simulink model "bh_compare_SM_vs_HAND_quad_and_spin_props"  (R2021b)
settings: Solver=ode23t  StartTime=0.0  StopTime=200  FixedStep=0.001  RelTol=1e-5  EnableMultiTasking=on
undefined symbols (not defined in the file or in its folder): P_elec, P_mot, P_one_prop, P_rot, P_veh, P_veh_no_props, sigbuilder_block, X, xme_dot_0, Y, Z
libraries: fl_lib x85, simulink_extras x40, nesl_utility x35, slpidlib x24, bh_6dof_LIBRARY x24, sm_lib x23, fl_ps_legacy_lib x7, simulink x2
(part 2 of 6)

== system bh_compare_SM_vs_HAND_quad_and_spin_props/XYZ CMD_LIMITS1 ==
  XYZ_in : Inport
  Bus Creator : BusCreator  Inputs=3
  Demux : Demux  Outputs=2
  Demux1 : Demux  Outputs=2
  Mux1 : Mux  Inputs=2
  Mux2 : Mux  Inputs=2
  Mux3 : Mux  Inputs=2
  Mux4 : Mux  Inputs=3
  Rate Limiter : RateLimiter  RisingSlewLimit=2  FallingSlewLimit=-2
      settings: AttributesFormatString=|
      | Rising_rate = %<RisingSlewLimit>
      | Falling_rate = %<FallingSlewLimit>
  Rate Limiter1 : RateLimiter  RisingSlewLimit=3  FallingSlewLimit=-3
      settings: AttributesFormatString=|
      | Rising_rate = %<RisingSlewLimit>
      | Falling_rate = %<FallingSlewLimit>
  Rate Limiter2 : RateLimiter  RisingSlewLimit=3  FallingSlewLimit=-3
      settings: AttributesFormatString=|
      | Rising_rate = %<RisingSlewLimit>
      | Falling_rate = %<FallingSlewLimit>
  Reshape : Reshape  OutputDimensionality=Column vector (2-D)
  Saturation : Saturate  UpperLimit=500  LowerLimit=0
      settings: AttributesFormatString=|
      | MAX =    %<UpperLimit>
      | MIN = %<LowerLimit>
  Saturation1 : Saturate  UpperLimit=500  LowerLimit=-500
      settings: AttributesFormatString=|
      | MAX =    %<UpperLimit>
      | MIN = %<LowerLimit>
  Saturation2 : Saturate  UpperLimit=500  LowerLimit=-500
      settings: AttributesFormatString=|
      | MAX =    %<UpperLimit>
      | MIN = %<LowerLimit>
  Selector : Selector  InputPortWidth=3  IndexOptions=Index vector (dialog)  Indices=3  OutputSizes=1
  Selector1 : Selector  InputPortWidth=3  IndexOptions=Index vector (dialog)  Indices=[1 2]  OutputSizes=1
  Unit Delay : UnitDelay  SampleTime=0.01  HasFrameUpgradeWarning=on
  Unit Delay1 : UnitDelay  SampleTime=0.01  HasFrameUpgradeWarning=on
  ZXY_LIMITED : Scope  NumInputPorts=3
  prefilter : Subsystem  Commented=on  mask(Derivative Estimation){wn=2*pi*0.5, p=1}
      mask prompts: wn "Natural frequency, wn (rad/sec)"; p "Damping ratio, p"
      mask help:
      | A simple derivative estimator using a 2nd order representation between input and output.
      |
      | The integrators use a discrete FORWARd Euler rule, and a sample time needs to be specified.
      mask init:
      | str1 = sprintf('wn = %.2f', wn);
      | str2 = sprintf('p  = %.2f', p);
      | %str3 = sprintf('dt = %.2f', dt);
      | %str = char(str1,str2,str3);
      | %str3 = sprintf('dt = %.2f', dt);
      | str = char(str1,str2);
      mask Display: disp(str)
  XYZ : Outport  VectorParamsAs1DForOutWhenUnconnected=off
  CMD_BUS : Outport  Port=2  VectorParamsAs1DForOutWhenUnconnected=off
  wires:
  Selector1/1 -> Demux1/1, Unit Delay1/1
  Demux/1 -> Rate Limiter1/1
  Demux/2 -> Rate Limiter2/1
  Saturation1/1 -> [X]
  Saturation2/1 -> [Y]
  Mux4/1 -> Reshape/1
  Selector/1 -> Mux1/1, Unit Delay/1
  Rate Limiter/1 -> Saturation/1
  Unit Delay/1 -> Rate Limiter/1
  Unit Delay1/1 -> Demux/1
  Rate Limiter1/1 -> Saturation1/1
  Rate Limiter2/1 -> Saturation2/1
  [X] -> Mux4/1
  [Y] -> Mux4/2
  [Z] -> Mux4/3
  Saturation/1 -> [Z]
  [Z] -> Mux1/2
  [Y] -> Mux3/2
  Demux1/1 -> Mux2/1
  Demux1/2 -> Mux3/1
  [X] -> Mux2/2
  Mux1/1 -> ZXY_LIMITED/1  "Z"
  Mux2/1 -> ZXY_LIMITED/2  "X"
  Mux3/1 -> ZXY_LIMITED/3  "Y"
  Bus Creator/1 -> CMD_BUS/1
  [Y] -> Bus Creator/2  "Y"
  [X] -> Bus Creator/1  "X"
  [Z] -> Bus Creator/3  "Z"
  Reshape/1 -> XYZ/1
  XYZ_in/1 -> Selector1/1, Selector/1

== system bh_compare_SM_vs_HAND_quad_and_spin_props/a_circle1 ==
  Clock : Clock
  Clock1 : Clock
  Constant4 : Constant  Value=0  VectorParams1D=off
  Constant5 : Constant  Value=20  VectorParams1D=off
  Constant6 : Constant  Value=2  VectorParams1D=off
  Constant7 : Constant  VectorParams1D=off
  Constant8 : Constant  Value=0.05  VectorParams1D=off
  MATLAB Function : MATLAB Function  TreatAsAtomicUnit=on
  Mux1 : Mux  Inputs=3
  Reshape1 : Reshape  OutputDimensionality=Column vector (2-D)
  Reshape2 : Reshape  OutputDimensionality=Column vector (2-D)
  Signal Builder : Subsystem  Tag=STV Subsys  LoadFcn=sigbuilder_block('load');  StartFcn=sigbuilder_block('start');  StopFcn=sigbuilder_block('stop');  ClipboardFcn=sigbuilder_block('clipboard');  mask(Sigbuilder block){tuvar=[0:10]}
      mask help: Simulink:masks:SigbuilderBlock_MD
      mask init:
      | if ~strcmp(get_param(bdroot(gcbh),'SimulationStatus'),'stopped') tuvar = sigbuilder_block('maskInit'); end
      settings: CopyFcn=sigbuilder_block('copy');  DeleteFcn=sigbuilder_block('delete');  ModelCloseFcn=sigbuilder_block('modelClose');  PreSaveFcn=sigbuilder_block('preSave');  PauseFcn=sigbuilder_block('pause');  ContinueFcn=sigbuilder_block('continue');  NameChangeFcn=sigbuilder_block('namechange');  OpenFcn=sigbuilder_block('open',[437.6 199.2 550.4 400 ]);  CloseFcn=sigbuilder_block('close');
      mask Display: plot(0, 0, 100, 100,[2, 2, 32, 32, 2], [68, 8, 8, 68, 68],[32, 2], [38, 38], [32, 19, 2],[53, 60, 44], [32, 17, 17, 2],[16, 16, 31, 31]);txt = getActiveGroup(gcbh);text(2, 100, txt,'verticalAlignment', 'top');
  Subsystem : Subsystem
  Switch : Switch  Criteria=u2 > Threshold  Threshold=20
  Out1 : Outport  VectorParamsAs1DForOutWhenUnconnected=off
  wires:
  Switch/1 -> Out1/1
  MATLAB Function/1(XYZ) -> Reshape2/1
  Constant6/1 -> MATLAB Function/3(RADIUS)
  Constant7/1 -> MATLAB Function/4(ztgt)
  Subsystem/1(w_rad_psec) -> MATLAB Function/5(w)
  Constant5/1 -> MATLAB Function/2(t_to_start)
  Reshape1/1 -> Switch/3
  Constant4/1 -> Mux1/2
  Signal Builder/1(Signal 1) -> Mux1/1
  Signal Builder/2(Signal 2) -> Mux1/3
  Mux1/1 -> Reshape1/1
  Clock/1 -> Switch/2
  Clock1/1 -> MATLAB Function/1(t_clock)
  Constant8/1 -> Subsystem/1(RPS)
  Reshape2/1 -> Switch/1

== system bh_compare_SM_vs_HAND_quad_and_spin_props/CONT_SYS Force_Moment_CMDS/FM_CMD_LIMITS ==
  T_CMD : Inport
  TQ_Roll : Inport  Port=2
  TQ_Pitch : Inport  Port=3
  TQ_Yaw : Inport  Port=4
  Mux : Mux
  Saturation : Saturate  UpperLimit=4*P_one_prop.thrust_max  LowerLimit=0
      settings: AttributesFormatString=|
      | MAX =    %<UpperLimit>
      | MIN = %<LowerLimit>
  Saturation1 : Saturate  UpperLimit=2*P_one_prop.TQ_max  LowerLimit=-2*P_one_prop.TQ_max
      settings: AttributesFormatString=|
      | MAX =    %<UpperLimit>
      | MIN = %<LowerLimit>
  Saturation2 : Saturate  UpperLimit="P_one_prop.thrust_max *  P_veh.L_CG_to_mot"  LowerLimit="-P_one_prop.thrust_max *  P_veh.L_CG_to_mot"
      settings: AttributesFormatString=|
      | MAX =    %<UpperLimit>
      | MIN = %<LowerLimit>
  Saturation3 : Saturate  UpperLimit="P_one_prop.thrust_max *  P_veh.L_CG_to_mot"  LowerLimit="-P_one_prop.thrust_max *  P_veh.L_CG_to_mot"
      settings: AttributesFormatString=|
      | MAX =    %<UpperLimit>
      | MIN = %<LowerLimit>
  THRUST : Outport  VectorParamsAs1DForOutWhenUnconnected=off
  TQ_Roll_X : Outport  Port=2  VectorParamsAs1DForOutWhenUnconnected=off
  TQ_Pitch_Y : Outport  Port=3  VectorParamsAs1DForOutWhenUnconnected=off
  TQ_Yaw_Z : Outport  Port=4  VectorParamsAs1DForOutWhenUnconnected=off
  CMD_VEC : Outport  Port=5  VectorParamsAs1DForOutWhenUnconnected=off
  wires:
  TQ_Yaw/1 -> Saturation1/1
  T_CMD/1 -> Saturation/1
  TQ_Pitch/1 -> Saturation2/1
  TQ_Roll/1 -> Saturation3/1
  Saturation/1 -> [THRUST], THRUST/1
  Saturation3/1 -> [TQ_Roll_X], TQ_Roll_X/1
  Saturation2/1 -> [TQ_Pitch_Y], TQ_Pitch_Y/1
  Saturation1/1 -> [TQ_Yaw_Z], TQ_Yaw_Z/1
  Mux/1 -> CMD_VEC/1
  [THRUST] -> Mux/1
  [TQ_Roll_X] -> Mux/2
  [TQ_Pitch_Y] -> Mux/3
  [TQ_Yaw_Z] -> Mux/4

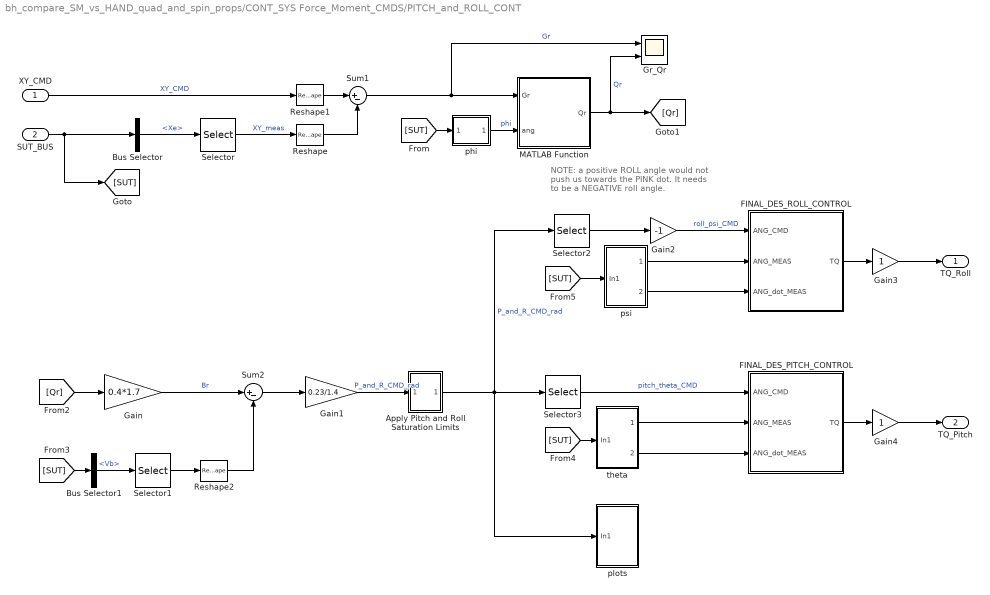
== system bh_compare_SM_vs_HAND_quad_and_spin_props/CONT_SYS Force_Moment_CMDS/PITCH_and_ROLL_CONT ==
  note: NOTE:  a positive ROLL angle would
      | not push us towards the PINK dot.  It
      | needs to be a NEGATIVE roll angle.
  XY_CMD : Inport
  SUT_BUS : Inport  Port=2
  Apply Pitch and Roll Saturation Limits : Subsystem
  Bus Selector : BusSelector  OutputSignals=Xe
  Bus Selector1 : BusSelector  OutputSignals=Vb
  FINAL_DES_PITCH_CONTROL : Subsystem
  FINAL_DES_ROLL_CONTROL : Subsystem
  Gain : Gain  Gain=0.4*1.7
  Gain1 : Gain  Gain=0.23/1.4
  Gain2 : Gain  Gain=-1
  Gain3 : Gain
  Gain4 : Gain
  Gr_Qr : Scope  NumInputPorts=2
  MATLAB Function : MATLAB Function  TreatAsAtomicUnit=on
  Reshape : Reshape  OutputDimensionality=Column vector (2-D)
  Reshape1 : Reshape  OutputDimensionality=Column vector (2-D)
  Reshape2 : Reshape  OutputDimensionality=Column vector (2-D)
  Selector : Selector  InputPortWidth=3  IndexOptions=Index vector (dialog)  Indices=[1 2]  OutputSizes=1
  Selector1 : Selector  InputPortWidth=3  IndexOptions=Index vector (dialog)  Indices=[1 2]  OutputSizes=1
  Selector2 : Selector  InputPortWidth=2  IndexOptions=Index vector (dialog)  Indices=2  OutputSizes=1
  Selector3 : Selector  InputPortWidth=2  IndexOptions=Index vector (dialog)  Indices=1  OutputSizes=1
  Sum1 : Sum  Inputs=|+-
  Sum2 : Sum  Inputs=|+-
  phi : Subsystem
  plots : Subsystem
  psi : Subsystem
  theta : Subsystem
  TQ_Roll : Outport  VectorParamsAs1DForOutWhenUnconnected=off
  TQ_Pitch : Outport  Port=2  VectorParamsAs1DForOutWhenUnconnected=off
  wires:
  Bus Selector/1 -> Selector/1  "<Xe>"
  Selector/1 -> Reshape/1  "XY_meas"
  SUT_BUS/1 -> Bus Selector/1, [SUT]
  XY_CMD/1 -> Reshape1/1  "XY_CMD"
  Reshape1/1 -> Sum1/1
  Reshape/1 -> Sum1/2
  Sum1/1 -> Gr_Qr/1, MATLAB Function/1(Gr)  "Gr"
  [SUT] -> phi/1(In1)
  phi/1(Out1) -> MATLAB Function/2(ang)  "phi"
  MATLAB Function/1(Qr) -> Gr_Qr/2, [Qr]  "Qr"
  [Qr] -> Gain/1
  Gain/1 -> Sum2/1  "Br"
  Bus Selector1/1 -> Selector1/1  "<Vb>"
  [SUT] -> Bus Selector1/1
  Selector1/1 -> Reshape2/1
  Reshape2/1 -> Sum2/2
  Sum2/1 -> Gain1/1
  [SUT] -> theta/1(In1)
  theta/1(Out1) -> FINAL_DES_PITCH_CONTROL/2(ANG_MEAS)
  theta/2(Out2) -> FINAL_DES_PITCH_CONTROL/3(ANG_dot_MEAS)
  Selector3/1 -> FINAL_DES_PITCH_CONTROL/1(ANG_CMD)  "pitch_theta_CMD"
  FINAL_DES_PITCH_CONTROL/1(TQ) -> Gain4/1
  Gain1/1 -> Apply Pitch and Roll Saturation Limits/1(In1)  "P_and_R_CMD_rad"
  Selector2/1 -> Gain2/1
  psi/1(Out1) -> FINAL_DES_ROLL_CONTROL/2(ANG_MEAS)
  psi/2(Out2) -> FINAL_DES_ROLL_CONTROL/3(ANG_dot_MEAS)
  [SUT] -> psi/1(In1)
  FINAL_DES_ROLL_CONTROL/1(TQ) -> Gain3/1
  Gain2/1 -> FINAL_DES_ROLL_CONTROL/1(ANG_CMD)  "roll_psi_CMD"
  Apply Pitch and Roll Saturation Limits/1(Out1) -> plots/1(In1), Selector3/1, Selector2/1  "P_and_R_CMD_rad"
  Gain3/1 -> TQ_Roll/1
  Gain4/1 -> TQ_Pitch/1

== system bh_compare_SM_vs_HAND_quad_and_spin_props/CONT_SYS Force_Moment_CMDS/YAW_CONT ==
  Yaw_CMD : Inport
  SUT_BUS : Inport  Port=2
  Bus Selector3 : BusSelector  OutputSignals=phi_theta_psi
  Bus Selector4 : BusSelector  OutputSignals=DOT_phi_theta_psi
  FINAL_DES_YAW_CONTROL_SYSTEM : Subsystem
  Selector2 : Selector  InputPortWidth=3  IndexOptions=Index vector (dialog)  Indices=1  OutputSizes=1
  Selector3 : Selector  InputPortWidth=3  IndexOptions=Index vector (dialog)  Indices=1  OutputSizes=1
  TQ_Yaw : Outport  VectorParamsAs1DForOutWhenUnconnected=off
  wires:
  Selector2/1 -> FINAL_DES_YAW_CONTROL_SYSTEM/2(YAW_MEAS)
  Yaw_CMD/1 -> FINAL_DES_YAW_CONTROL_SYSTEM/1(YAW_CMD)
  Selector3/1 -> FINAL_DES_YAW_CONTROL_SYSTEM/3(YAW_dot_MEAS)
  FINAL_DES_YAW_CONTROL_SYSTEM/1(TQ_YAW) -> TQ_Yaw/1  "TQ_Z_YAW"
  Bus Selector4/1 -> Selector3/1  "<DOT_phi_theta_psi>"
  Bus Selector3/1 -> Selector2/1  "<phi_theta_psi>"
  SUT_BUS/1 -> Bus Selector4/1, Bus Selector3/1

== system bh_compare_SM_vs_HAND_quad_and_spin_props/CONT_SYS Force_Moment_CMDS/Z_CONT ==
  Ze_CMD : Inport
  SUT_BUS : Inport  Port=2
  Bus Selector : BusSelector  OutputSignals=Xe
  Bus Selector2 : BusSelector  OutputSignals=Ve
  FINAL_DES_ALTITUDE_CONTROL_SYSTEM : Subsystem
  Selector : Selector  InputPortWidth=3  IndexOptions=Index vector (dialog)  Indices=3  OutputSizes=1
  Selector1 : Selector  InputPortWidth=3  IndexOptions=Index vector (dialog)  Indices=3  OutputSizes=1
  Ze_to_Altitude : bh_6dof_LIBRARY/MODELS/Ze_to_Altitude  SystemSampleTime=-1  VariantActivationTime=update diagram  Latency=0  AutoFrameSizeCalculation=off
  THRUST : Outport  VectorParamsAs1DForOutWhenUnconnected=off
  wires:
  Selector1/1 -> FINAL_DES_ALTITUDE_CONTROL_SYSTEM/3(Ze_dot_MEAS)
  Ze_to_Altitude/1 -> FINAL_DES_ALTITUDE_CONTROL_SYSTEM/2(Ze_MEAS)
  FINAL_DES_ALTITUDE_CONTROL_SYSTEM/1(THRUST) -> THRUST/1
  SUT_BUS/1 -> Bus Selector2/1, Bus Selector/1
  Ze_CMD/1 -> FINAL_DES_ALTITUDE_CONTROL_SYSTEM/1(Ze_CMD)
  Bus Selector2/1 -> Selector1/1  "<Ve>"
  Bus Selector/1 -> Selector/1  "<Xe>"
  Selector/1 -> Ze_to_Altitude/1

== system bh_compare_SM_vs_HAND_quad_and_spin_props/CONT_SYS Force_Moment_CMDS1/FM_CMD_LIMITS ==
  T_CMD : Inport
  TQ_Roll : Inport  Port=2
  TQ_Pitch : Inport  Port=3
  TQ_Yaw : Inport  Port=4
  Mux : Mux
  Saturation : Saturate  UpperLimit=4*P_one_prop.thrust_max  LowerLimit=0
      settings: AttributesFormatString=|
      | MAX =    %<UpperLimit>
      | MIN = %<LowerLimit>
  Saturation1 : Saturate  UpperLimit=2*P_one_prop.TQ_max  LowerLimit=-2*P_one_prop.TQ_max
      settings: AttributesFormatString=|
      | MAX =    %<UpperLimit>
      | MIN = %<LowerLimit>
  Saturation2 : Saturate  UpperLimit="P_one_prop.thrust_max *  P_veh.L_CG_to_mot"  LowerLimit="-P_one_prop.thrust_max *  P_veh.L_CG_to_mot"
      settings: AttributesFormatString=|
      | MAX =    %<UpperLimit>
      | MIN = %<LowerLimit>
  Saturation3 : Saturate  UpperLimit="P_one_prop.thrust_max *  P_veh.L_CG_to_mot"  LowerLimit="-P_one_prop.thrust_max *  P_veh.L_CG_to_mot"
      settings: AttributesFormatString=|
      | MAX =    %<UpperLimit>
      | MIN = %<LowerLimit>
  THRUST : Outport  VectorParamsAs1DForOutWhenUnconnected=off
  TQ_Roll_X : Outport  Port=2  VectorParamsAs1DForOutWhenUnconnected=off
  TQ_Pitch_Y : Outport  Port=3  VectorParamsAs1DForOutWhenUnconnected=off
  TQ_Yaw_Z : Outport  Port=4  VectorParamsAs1DForOutWhenUnconnected=off
  CMD_VEC : Outport  Port=5  VectorParamsAs1DForOutWhenUnconnected=off
  wires:
  TQ_Yaw/1 -> Saturation1/1
  T_CMD/1 -> Saturation/1
  TQ_Pitch/1 -> Saturation2/1
  TQ_Roll/1 -> Saturation3/1
  Saturation/1 -> [THRUST], THRUST/1
  Saturation3/1 -> [TQ_Roll_X], TQ_Roll_X/1
  Saturation2/1 -> [TQ_Pitch_Y], TQ_Pitch_Y/1
  Saturation1/1 -> [TQ_Yaw_Z], TQ_Yaw_Z/1
  Mux/1 -> CMD_VEC/1
  [THRUST] -> Mux/1
  [TQ_Roll_X] -> Mux/2
  [TQ_Pitch_Y] -> Mux/3
  [TQ_Yaw_Z] -> Mux/4

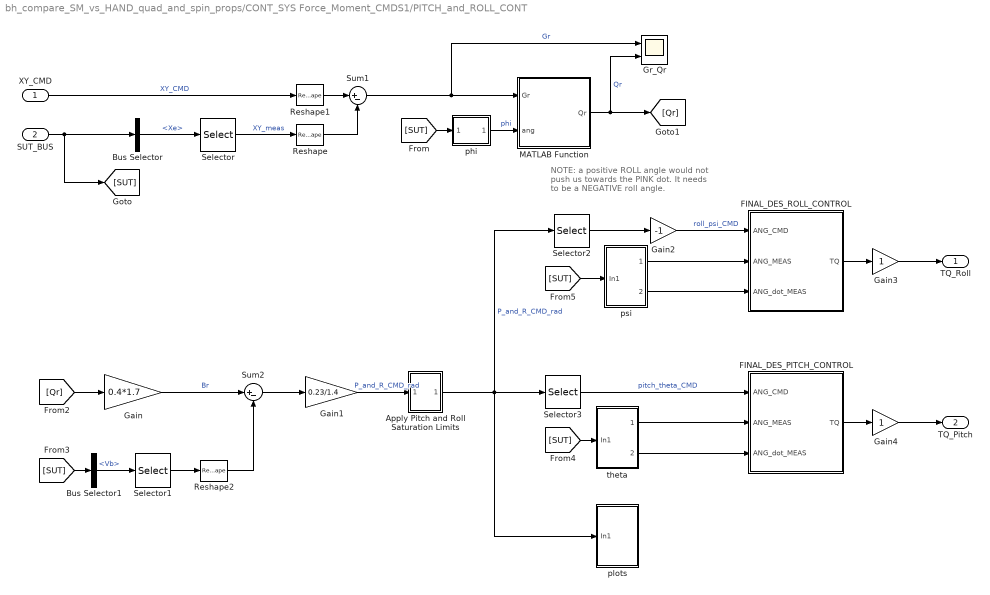
== system bh_compare_SM_vs_HAND_quad_and_spin_props/CONT_SYS Force_Moment_CMDS1/PITCH_and_ROLL_CONT ==
  note: NOTE:  a positive ROLL angle would
      | not push us towards the PINK dot.  It
      | needs to be a NEGATIVE roll angle.
  XY_CMD : Inport
  SUT_BUS : Inport  Port=2
  Apply Pitch and Roll Saturation Limits : Subsystem
  Bus Selector : BusSelector  OutputSignals=Xe
  Bus Selector1 : BusSelector  OutputSignals=Vb
  FINAL_DES_PITCH_CONTROL : Subsystem
  FINAL_DES_ROLL_CONTROL : Subsystem
  Gain : Gain  Gain=0.4*1.7
  Gain1 : Gain  Gain=0.23/1.4
  Gain2 : Gain  Gain=-1
  Gain3 : Gain
  Gain4 : Gain
  Gr_Qr : Scope  NumInputPorts=2
  MATLAB Function : MATLAB Function  TreatAsAtomicUnit=on
  Reshape : Reshape  OutputDimensionality=Column vector (2-D)
  Reshape1 : Reshape  OutputDimensionality=Column vector (2-D)
  Reshape2 : Reshape  OutputDimensionality=Column vector (2-D)
  Selector : Selector  InputPortWidth=3  IndexOptions=Index vector (dialog)  Indices=[1 2]  OutputSizes=1
  Selector1 : Selector  InputPortWidth=3  IndexOptions=Index vector (dialog)  Indices=[1 2]  OutputSizes=1
  Selector2 : Selector  InputPortWidth=2  IndexOptions=Index vector (dialog)  Indices=2  OutputSizes=1
  Selector3 : Selector  InputPortWidth=2  IndexOptions=Index vector (dialog)  Indices=1  OutputSizes=1
  Sum1 : Sum  Inputs=|+-
  Sum2 : Sum  Inputs=|+-
  phi : Subsystem
  plots : Subsystem
  psi : Subsystem
  theta : Subsystem
  TQ_Roll : Outport  VectorParamsAs1DForOutWhenUnconnected=off
  TQ_Pitch : Outport  Port=2  VectorParamsAs1DForOutWhenUnconnected=off
  wires:
  Bus Selector/1 -> Selector/1  "<Xe>"
  Selector/1 -> Reshape/1  "XY_meas"
  SUT_BUS/1 -> Bus Selector/1, [SUT]
  XY_CMD/1 -> Reshape1/1  "XY_CMD"
  Reshape1/1 -> Sum1/1
  Reshape/1 -> Sum1/2
  Sum1/1 -> Gr_Qr/1, MATLAB Function/1(Gr)  "Gr"
  [SUT] -> phi/1(In1)
  phi/1(Out1) -> MATLAB Function/2(ang)  "phi"
  MATLAB Function/1(Qr) -> Gr_Qr/2, [Qr]  "Qr"
  [Qr] -> Gain/1
  Gain/1 -> Sum2/1  "Br"
  Bus Selector1/1 -> Selector1/1  "<Vb>"
  [SUT] -> Bus Selector1/1
  Selector1/1 -> Reshape2/1
  Reshape2/1 -> Sum2/2
  Sum2/1 -> Gain1/1
  [SUT] -> theta/1(In1)
  theta/1(Out1) -> FINAL_DES_PITCH_CONTROL/2(ANG_MEAS)
  theta/2(Out2) -> FINAL_DES_PITCH_CONTROL/3(ANG_dot_MEAS)
  Selector3/1 -> FINAL_DES_PITCH_CONTROL/1(ANG_CMD)  "pitch_theta_CMD"
  FINAL_DES_PITCH_CONTROL/1(TQ) -> Gain4/1
  Gain1/1 -> Apply Pitch and Roll Saturation Limits/1(In1)  "P_and_R_CMD_rad"
  Selector2/1 -> Gain2/1
  psi/1(Out1) -> FINAL_DES_ROLL_CONTROL/2(ANG_MEAS)
  psi/2(Out2) -> FINAL_DES_ROLL_CONTROL/3(ANG_dot_MEAS)
  [SUT] -> psi/1(In1)
  FINAL_DES_ROLL_CONTROL/1(TQ) -> Gain3/1
  Gain2/1 -> FINAL_DES_ROLL_CONTROL/1(ANG_CMD)  "roll_psi_CMD"
  Apply Pitch and Roll Saturation Limits/1(Out1) -> plots/1(In1), Selector3/1, Selector2/1  "P_and_R_CMD_rad"
  Gain3/1 -> TQ_Roll/1
  Gain4/1 -> TQ_Pitch/1

== system bh_compare_SM_vs_HAND_quad_and_spin_props/CONT_SYS Force_Moment_CMDS1/YAW_CONT ==
  Yaw_CMD : Inport
  SUT_BUS : Inport  Port=2
  Bus Selector3 : BusSelector  OutputSignals=phi_theta_psi
  Bus Selector4 : BusSelector  OutputSignals=DOT_phi_theta_psi
  FINAL_DES_YAW_CONTROL_SYSTEM : Subsystem
  Selector2 : Selector  InputPortWidth=3  IndexOptions=Index vector (dialog)  Indices=1  OutputSizes=1
  Selector3 : Selector  InputPortWidth=3  IndexOptions=Index vector (dialog)  Indices=1  OutputSizes=1
  TQ_Yaw : Outport  VectorParamsAs1DForOutWhenUnconnected=off
  wires:
  Selector2/1 -> FINAL_DES_YAW_CONTROL_SYSTEM/2(YAW_MEAS)
  Yaw_CMD/1 -> FINAL_DES_YAW_CONTROL_SYSTEM/1(YAW_CMD)
  Selector3/1 -> FINAL_DES_YAW_CONTROL_SYSTEM/3(YAW_dot_MEAS)
  FINAL_DES_YAW_CONTROL_SYSTEM/1(TQ_YAW) -> TQ_Yaw/1  "TQ_Z_YAW"
  Bus Selector4/1 -> Selector3/1  "<DOT_phi_theta_psi>"
  Bus Selector3/1 -> Selector2/1  "<phi_theta_psi>"
  SUT_BUS/1 -> Bus Selector4/1, Bus Selector3/1

== system bh_compare_SM_vs_HAND_quad_and_spin_props/CONT_SYS Force_Moment_CMDS1/Z_CONT ==
  Ze_CMD : Inport
  SUT_BUS : Inport  Port=2
  Bus Selector : BusSelector  OutputSignals=Xe
  Bus Selector2 : BusSelector  OutputSignals=Ve
  FINAL_DES_ALTITUDE_CONTROL_SYSTEM : Subsystem
  Selector : Selector  InputPortWidth=3  IndexOptions=Index vector (dialog)  Indices=3  OutputSizes=1
  Selector1 : Selector  InputPortWidth=3  IndexOptions=Index vector (dialog)  Indices=3  OutputSizes=1
  Ze_to_Altitude : bh_6dof_LIBRARY/MODELS/Ze_to_Altitude  SystemSampleTime=-1  VariantActivationTime=update diagram  Latency=0  AutoFrameSizeCalculation=off
  THRUST : Outport  VectorParamsAs1DForOutWhenUnconnected=off
  wires:
  Selector1/1 -> FINAL_DES_ALTITUDE_CONTROL_SYSTEM/3(Ze_dot_MEAS)
  Ze_to_Altitude/1 -> FINAL_DES_ALTITUDE_CONTROL_SYSTEM/2(Ze_MEAS)
  FINAL_DES_ALTITUDE_CONTROL_SYSTEM/1(THRUST) -> THRUST/1
  SUT_BUS/1 -> Bus Selector2/1, Bus Selector/1
  Ze_CMD/1 -> FINAL_DES_ALTITUDE_CONTROL_SYSTEM/1(Ze_CMD)
  Bus Selector2/1 -> Selector1/1  "<Ve>"
  Bus Selector/1 -> Selector/1  "<Xe>"
  Selector/1 -> Ze_to_Altitude/1

== system bh_compare_SM_vs_HAND_quad_and_spin_props/CONT_SYS W_MOT_CMDS/MOTOR_sys ==
  w_CMD : Inport
  Demux : Demux
  MOTOR_1 : Subsystem
      mask Display: image('bh_PIC_MOTOR.jpg');
  MOTOR_2 : Subsystem
      mask Display: image('bh_PIC_MOTOR.jpg');
  MOTOR_3 : Subsystem
      mask Display: image('bh_PIC_MOTOR.jpg');
  MOTOR_4 : Subsystem
      mask Display: image('bh_PIC_MOTOR.jpg');
  Mux : Mux
  w CMD vs Actual : Scope  NumInputPorts=4
  w_MUX : Subsystem
  w : Outport  VectorParamsAs1DForOutWhenUnconnected=off
  wires:
  MOTOR_4/1(w) -> Mux/4
  MOTOR_3/1(w) -> Mux/3
  MOTOR_2/1(w) -> Mux/2
  MOTOR_1/1(w) -> Mux/1
  Demux/1 -> MOTOR_1/1(w_CMD)
  Demux/2 -> MOTOR_2/1(w_CMD)
  Demux/3 -> MOTOR_3/1(w_CMD)
  Demux/4 -> MOTOR_4/1(w_CMD)
  w_CMD/1 -> [W_CMD], Demux/1
  w_MUX/4(w4) -> w CMD vs Actual/4
  w_MUX/2(w2) -> w CMD vs Actual/2
  w_MUX/3(w3) -> w CMD vs Actual/3
  w_MUX/1(w1) -> w CMD vs Actual/1
  [W_CMD] -> w_MUX/1(W_CMD)
  Mux/1 -> w_MUX/2(W), w/1

== system bh_compare_SM_vs_HAND_quad_and_spin_props/CONT_SYS W_MOT_CMDS/SIGN_CONVENTIONS ==

== system bh_compare_SM_vs_HAND_quad_and_spin_props/CONT_SYS W_MOT_CMDS/W2_checker ==
  w2_CMD : Inport
  Assertion{,1..3} (4 alike) : Assertion
  Compare To Constant : simulink/Logic and Bit Operations/Compare To Constant  relop=>=  const=0  OutDataTypeStr=boolean
  Demux : Demux
  w2 : Outport  VectorParamsAs1DForOutWhenUnconnected=off
  wires:
  w2_CMD/1 -> w2/1, Compare To Constant/1
  Compare To Constant/1 -> Demux/1
  Demux/1 -> Assertion/1
  Demux/4 -> Assertion3/1
  Demux/3 -> Assertion2/1
  Demux/2 -> Assertion1/1

== system bh_compare_SM_vs_HAND_quad_and_spin_props/CONT_SYS W_MOT_CMDS2/PRE_FILTERS ==
  w_in : Inport
  Demux : Demux
  Mux : Mux
  Reshape2 : Reshape  OutputDimensionality=Column vector (2-D)
  Terminator{,1..3} (4 alike) : Terminator
  prefilter : Subsystem  mask(Derivative Estimation){wn=2*pi*5, p=1}
      mask prompts: wn "Natural frequency, wn (rad/sec)"; p "Damping ratio, p"
      mask help:
      | A simple derivative estimator using a 2nd order representation between input and output.
      |
      | The integrators use a discrete FORWARd Euler rule, and a sample time needs to be specified.
      mask init:
      | str1 = sprintf('wn = %.2f', wn);
      | str2 = sprintf('p  = %.2f', p);
      | %str3 = sprintf('dt = %.2f', dt);
      | %str = char(str1,str2,str3);
      | %str3 = sprintf('dt = %.2f', dt);
      | str = char(str1,str2);
      mask Display: disp(str)
  prefilter1 : Subsystem  mask(Derivative Estimation){wn=2*pi*5, p=1}
      mask prompts: wn "Natural frequency, wn (rad/sec)"; p "Damping ratio, p"
      mask help:
      | A simple derivative estimator using a 2nd order representation between input and output.
      |
      | The integrators use a discrete FORWARd Euler rule, and a sample time needs to be specified.
      mask init:
      | str1 = sprintf('wn = %.2f', wn);
      | str2 = sprintf('p  = %.2f', p);
      | %str3 = sprintf('dt = %.2f', dt);
      | %str = char(str1,str2,str3);
      | %str3 = sprintf('dt = %.2f', dt);
      | str = char(str1,str2);
      mask Display: disp(str)
  prefilter2 : Subsystem  mask(Derivative Estimation){wn=2*pi*5, p=1}
      mask prompts: wn "Natural frequency, wn (rad/sec)"; p "Damping ratio, p"
      mask help:
      | A simple derivative estimator using a 2nd order representation between input and output.
      |
      | The integrators use a discrete FORWARd Euler rule, and a sample time needs to be specified.
      mask init:
      | str1 = sprintf('wn = %.2f', wn);
      | str2 = sprintf('p  = %.2f', p);
      | %str3 = sprintf('dt = %.2f', dt);
      | %str = char(str1,str2,str3);
      | %str3 = sprintf('dt = %.2f', dt);
      | str = char(str1,str2);
      mask Display: disp(str)
  prefilter3 : Subsystem  mask(Derivative Estimation){wn=2*pi*5, p=1}
      mask prompts: wn "Natural frequency, wn (rad/sec)"; p "Damping ratio, p"
      mask help:
      | A simple derivative estimator using a 2nd order representation between input and output.
      |
      | The integrators use a discrete FORWARd Euler rule, and a sample time needs to be specified.
      mask init:
      | str1 = sprintf('wn = %.2f', wn);
      | str2 = sprintf('p  = %.2f', p);
      | %str3 = sprintf('dt = %.2f', dt);
      | %str = char(str1,str2,str3);
      | %str3 = sprintf('dt = %.2f', dt);
      | str = char(str1,str2);
      mask Display: disp(str)
  w CMD vs Actual : Scope  NumInputPorts=4
  w_MUX : Subsystem
  w : Outport  VectorParamsAs1DForOutWhenUnconnected=off
  wires:
  prefilter1/2(U_DOT) -> Terminator1/1
  prefilter/2(U_DOT) -> Terminator/1
  prefilter2/2(U_DOT) -> Terminator2/1
  prefilter3/2(U_DOT) -> Terminator3/1
  w_in/1 -> [W_CMD], Demux/1
  Demux/1 -> prefilter/1(U)
  Demux/2 -> prefilter1/1(U)
  Demux/3 -> prefilter2/1(U)
  Demux/4 -> prefilter3/1(U)
  prefilter/1(U_filt) -> Mux/1
  prefilter1/1(U_filt) -> Mux/2
  prefilter2/1(U_filt) -> Mux/3
  prefilter3/1(U_filt) -> Mux/4
  Mux/1 -> Reshape2/1
  Reshape2/1 -> w_MUX/2(W), w/1
  w_MUX/3(w3) -> w CMD vs Actual/3
  w_MUX/2(w2) -> w CMD vs Actual/2
  w_MUX/4(w4) -> w CMD vs Actual/4
  [W_CMD] -> w_MUX/1(W_CMD)
  w_MUX/1(w1) -> w CMD vs Actual/1

== system bh_compare_SM_vs_HAND_quad_and_spin_props/CONT_SYS W_MOT_CMDS2/SIGN_CONVENTIONS ==

== system bh_compare_SM_vs_HAND_quad_and_spin_props/CONT_SYS W_MOT_CMDS2/W2_checker ==
  w2_CMD : Inport
  Assertion{,1..3} (4 alike) : Assertion
  Compare To Constant : simulink/Logic and Bit Operations/Compare To Constant  relop=>=  const=0  OutDataTypeStr=boolean
  Demux : Demux
  w2 : Outport  VectorParamsAs1DForOutWhenUnconnected=off
  wires:
  w2_CMD/1 -> w2/1, Compare To Constant/1
  Compare To Constant/1 -> Demux/1
  Demux/1 -> Assertion/1
  Demux/4 -> Assertion3/1
  Demux/3 -> Assertion2/1
  Demux/2 -> Assertion1/1

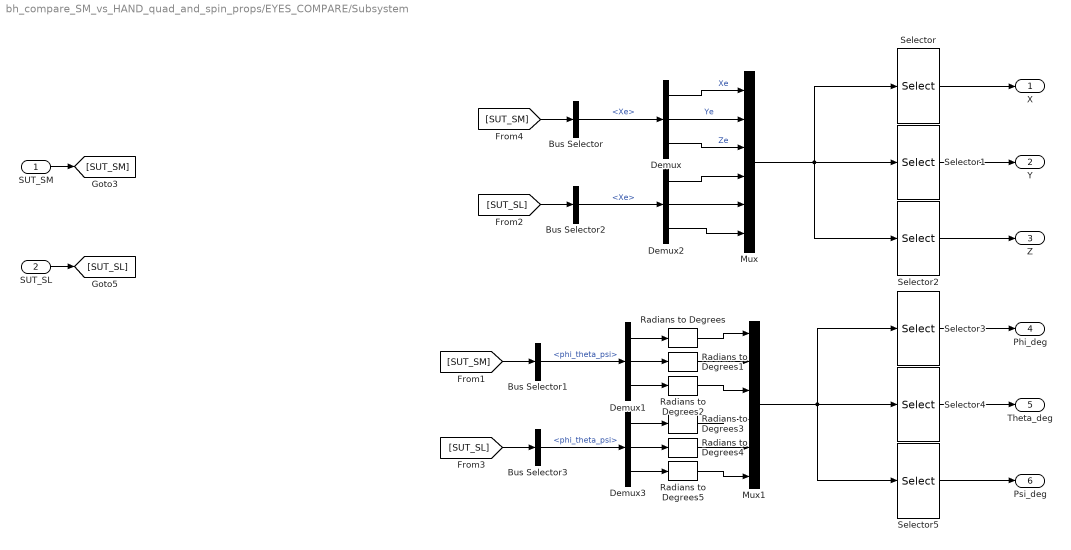
== system bh_compare_SM_vs_HAND_quad_and_spin_props/EYES_COMPARE/Subsystem ==
  SUT_SM : Inport
  SUT_SL : Inport  Port=2
  Bus Selector : BusSelector  OutputSignals=Xe
  Bus Selector1 : BusSelector  OutputSignals=phi_theta_psi
  Bus Selector2 : BusSelector  OutputSignals=Xe
  Bus Selector3 : BusSelector  OutputSignals=phi_theta_psi
  Demux{,1..3} (4 alike) : Demux  Outputs=3
  Mux : Mux  Inputs=6
  Mux1 : Mux  Inputs=6
  Radians to Degrees{,1..5} (6 alike) : simulink_extras/Transformations/Radians to Degrees
  Selector : Selector  InputPortWidth=6  IndexOptions=Index vector (dialog)  Indices=[1 4]  OutputSizes=1
  Selector1 : Selector  InputPortWidth=6  IndexOptions=Index vector (dialog)  Indices=[2 5]  OutputSizes=1
  Selector2 : Selector  InputPortWidth=6  IndexOptions=Index vector (dialog)  Indices=[3 6]  OutputSizes=1
  Selector3 : Selector  InputPortWidth=6  IndexOptions=Index vector (dialog)  Indices=[1 4]  OutputSizes=1
  Selector4 : Selector  InputPortWidth=6  IndexOptions=Index vector (dialog)  Indices=[2 5]  OutputSizes=1
  Selector5 : Selector  InputPortWidth=6  IndexOptions=Index vector (dialog)  Indices=[3 6]  OutputSizes=1
  X : Outport  VectorParamsAs1DForOutWhenUnconnected=off
  Y : Outport  Port=2  VectorParamsAs1DForOutWhenUnconnected=off
  Z : Outport  Port=3  VectorParamsAs1DForOutWhenUnconnected=off
  Phi_deg : Outport  Port=4  VectorParamsAs1DForOutWhenUnconnected=off
  Theta_deg : Outport  Port=5  VectorParamsAs1DForOutWhenUnconnected=off
  Psi_deg : Outport  Port=6  VectorParamsAs1DForOutWhenUnconnected=off
  wires:
  SUT_SL/1 -> [SUT_SL]
  SUT_SM/1 -> [SUT_SM]
  [SUT_SM] -> Bus Selector1/1
  Bus Selector1/1 -> Demux1/1  "<phi_theta_psi>"
  Bus Selector/1 -> Demux/1  "<Xe>"
  Demux1/2 -> Radians to Degrees1/1
  [SUT_SM] -> Bus Selector/1
  Demux1/1 -> Radians to Degrees/1
  Demux1/3 -> Radians to Degrees2/1
  [SUT_SL] -> Bus Selector2/1
  Bus Selector2/1 -> Demux2/1  "<Xe>"
  Demux3/1 -> Radians to Degrees3/1
  [SUT_SL] -> Bus Selector3/1
  Bus Selector3/1 -> Demux3/1  "<phi_theta_psi>"
  Demux3/2 -> Radians to Degrees4/1
  Demux3/3 -> Radians to Degrees5/1
  Demux2/2 -> Mux/5
  Demux2/3 -> Mux/6
  Demux2/1 -> Mux/4
  Demux/3 -> Mux/3  "Ze"
  Demux/2 -> Mux/2  "Ye"
  Demux/1 -> Mux/1  "Xe"
  Radians to Degrees5/1 -> Mux1/6
  Radians to Degrees4/1 -> Mux1/5
  Radians to Degrees3/1 -> Mux1/4
  Radians to Degrees2/1 -> Mux1/3
  Radians to Degrees1/1 -> Mux1/2
  Radians to Degrees/1 -> Mux1/1
  Mux/1 -> Selector/1, Selector2/1, Selector1/1
  Mux1/1 -> Selector5/1, Selector3/1, Selector4/1
  Selector2/1 -> Z/1
  Selector1/1 -> Y/1
  Selector/1 -> X/1
  Selector5/1 -> Psi_deg/1
  Selector4/1 -> Theta_deg/1
  Selector3/1 -> Phi_deg/1

== system bh_compare_SM_vs_HAND_quad_and_spin_props/EYES_PROP_and_VEH/THRUST_FUSE ==
  REF : Inport
  p1_b : Inport  Port=2
  p2_b : Inport  Port=3
  p3_b : Inport  Port=4
  p4_b : Inport  Port=5
  Bus Selector{,1..3} (4 alike) : BusSelector  OutputSignals=Thrust_on_veh
  Mux{,1..3} (4 alike) : Mux  Inputs=2
  Selector : Selector  InputPortWidth=4  IndexOptions=Index vector (dialog)  Indices=1  OutputSizes=1
  Selector1 : Selector  InputPortWidth=4  IndexOptions=Index vector (dialog)  Indices=2  OutputSizes=1
  Selector2 : Selector  InputPortWidth=4  IndexOptions=Index vector (dialog)  Indices=3  OutputSizes=1
  Selector3 : Selector  InputPortWidth=4  IndexOptions=Index vector (dialog)  Indices=4  OutputSizes=1
  Out1 : Outport  VectorParamsAs1DForOutWhenUnconnected=off
  Out2 : Outport  Port=2  VectorParamsAs1DForOutWhenUnconnected=off
  Out3 : Outport  Port=3  VectorParamsAs1DForOutWhenUnconnected=off
  Out4 : Outport  Port=4  VectorParamsAs1DForOutWhenUnconnected=off
  wires:
  Mux/1 -> Out4/1
  Mux1/1 -> Out3/1
  Mux2/1 -> Out2/1
  Mux3/1 -> Out1/1
  p1_b/1 -> Bus Selector/1
  Bus Selector/1 -> Mux3/2  "<Thrust_on_veh>"
  Selector/1 -> Mux3/1
  Selector1/1 -> Mux2/1
  Selector2/1 -> Mux1/1
  Selector3/1 -> Mux/1
  REF/1 -> Selector3/1, Selector2/1, Selector1/1, Selector/1
  p2_b/1 -> Bus Selector1/1
  Bus Selector1/1 -> Mux2/2  "<Thrust_on_veh>"
  p3_b/1 -> Bus Selector2/1
  Bus Selector2/1 -> Mux1/2  "<Thrust_on_veh>"
  p4_b/1 -> Bus Selector3/1
  Bus Selector3/1 -> Mux/2  "<Thrust_on_veh>"

== system bh_compare_SM_vs_HAND_quad_and_spin_props/EYES_PROP_and_VEH/TQ_FUSE ==
  REF : Inport
  p1_b : Inport  Port=2
  p2_b : Inport  Port=3
  p3_b : Inport  Port=4
  p4_b : Inport  Port=5
  Bus Selector{,1..3} (4 alike) : BusSelector  OutputSignals=Torque_on_veh
  Mux{,1..3} (4 alike) : Mux  Inputs=2
  Selector : Selector  InputPortWidth=4  IndexOptions=Index vector (dialog)  Indices=1  OutputSizes=1
  Selector1 : Selector  InputPortWidth=4  IndexOptions=Index vector (dialog)  Indices=2  OutputSizes=1
  Selector2 : Selector  InputPortWidth=4  IndexOptions=Index vector (dialog)  Indices=3  OutputSizes=1
  Selector3 : Selector  InputPortWidth=4  IndexOptions=Index vector (dialog)  Indices=4  OutputSizes=1
  Out1 : Outport  VectorParamsAs1DForOutWhenUnconnected=off
  Out2 : Outport  Port=2  VectorParamsAs1DForOutWhenUnconnected=off
  Out3 : Outport  Port=3  VectorParamsAs1DForOutWhenUnconnected=off
  Out4 : Outport  Port=4  VectorParamsAs1DForOutWhenUnconnected=off
  wires:
  Mux/1 -> Out4/1
  Mux1/1 -> Out3/1
  Mux2/1 -> Out2/1
  Mux3/1 -> Out1/1
  p1_b/1 -> Bus Selector/1
  Bus Selector/1 -> Mux3/2  "<Torque_on_veh>"
  Selector/1 -> Mux3/1
  Selector1/1 -> Mux2/1
  Selector2/1 -> Mux1/1
  Selector3/1 -> Mux/1
  REF/1 -> Selector3/1, Selector2/1, Selector1/1, Selector/1
  p2_b/1 -> Bus Selector1/1
  Bus Selector1/1 -> Mux2/2  "<Torque_on_veh>"
  p3_b/1 -> Bus Selector2/1
  Bus Selector2/1 -> Mux1/2  "<Torque_on_veh>"
  p4_b/1 -> Bus Selector3/1
  Bus Selector3/1 -> Mux/2  "<Torque_on_veh>"

== system bh_compare_SM_vs_HAND_quad_and_spin_props/EYES_PROP_and_VEH/w_FUSE ==
  REF : Inport
  p1_b : Inport  Port=2
  p2_b : Inport  Port=3
  p3_b : Inport  Port=4
  p4_b : Inport  Port=5
  Bus Selector{,1..3} (4 alike) : BusSelector  OutputSignals=w_prop
  Mux{,1..3} (4 alike) : Mux  Inputs=2
  Selector : Selector  InputPortWidth=4  IndexOptions=Index vector (dialog)  Indices=1  OutputSizes=1
  Selector1 : Selector  InputPortWidth=4  IndexOptions=Index vector (dialog)  Indices=2  OutputSizes=1
  Selector2 : Selector  InputPortWidth=4  IndexOptions=Index vector (dialog)  Indices=3  OutputSizes=1
  Selector3 : Selector  InputPortWidth=4  IndexOptions=Index vector (dialog)  Indices=4  OutputSizes=1
  Out1 : Outport  VectorParamsAs1DForOutWhenUnconnected=off
  Out2 : Outport  Port=2  VectorParamsAs1DForOutWhenUnconnected=off
  Out3 : Outport  Port=3  VectorParamsAs1DForOutWhenUnconnected=off
  Out4 : Outport  Port=4  VectorParamsAs1DForOutWhenUnconnected=off
  wires:
  Mux/1 -> Out4/1
  Mux1/1 -> Out3/1
  Mux2/1 -> Out2/1
  Mux3/1 -> Out1/1
  p1_b/1 -> Bus Selector/1
  Bus Selector/1 -> Mux3/2  "<w_prop>"
  Selector/1 -> Mux3/1
  Selector1/1 -> Mux2/1
  Selector2/1 -> Mux1/1
  Selector3/1 -> Mux/1
  REF/1 -> Selector3/1, Selector2/1, Selector1/1, Selector/1
  Bus Selector1/1 -> Mux2/2  "<w_prop>"
  p2_b/1 -> Bus Selector1/1
  Bus Selector2/1 -> Mux1/2  "<w_prop>"
  p3_b/1 -> Bus Selector2/1
  Bus Selector3/1 -> Mux/2  "<w_prop>"
  p4_b/1 -> Bus Selector3/1

== system bh_compare_SM_vs_HAND_quad_and_spin_props/MODEL_SYS/SIGN_CONVENTIONS ==

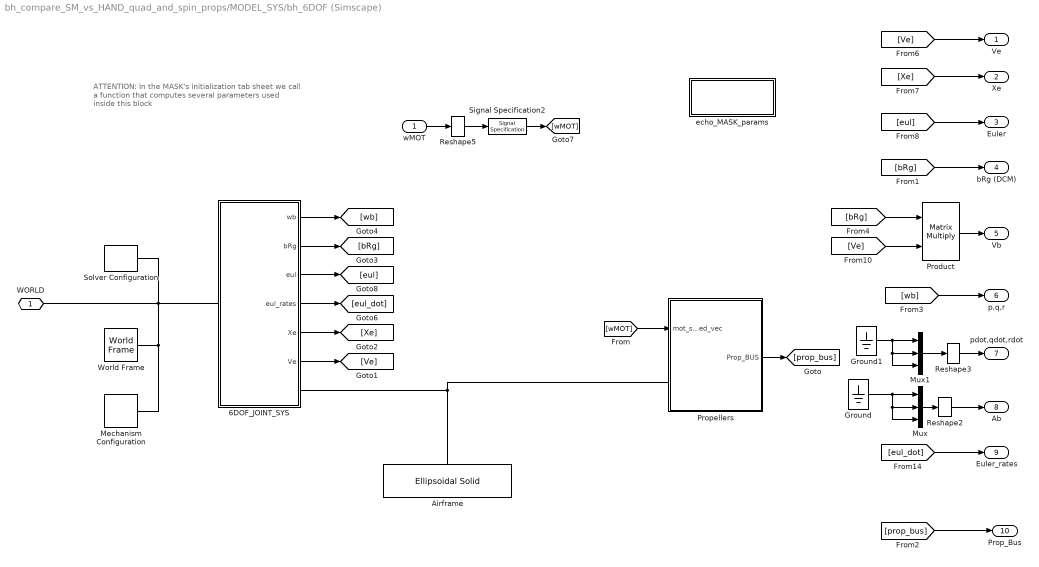
== system bh_compare_SM_vs_HAND_quad_and_spin_props/MODEL_SYS/bh_6DOF (Simscape) ==
  note: ATTENTION:
      | In the MASK's initialization tab sheet
      | we call a function that computes several parameters
      | used inside this block
  wMOT : Inport
  6DOF_JOINT_SYS : Subsystem
  Airframe : sm_lib/Body Elements/Ellipsoidal Solid  GraphicAmbientColor=[0.15 0.15 0.15 1.0]  BasedOnType=Density  CenterOfMass=[0 0 0]  CenterOfMassUnits=m  GraphicDiffuseColor=[0.5 0.5 0.5]  Density=1000  DensityUnits=kg/(m^3)  DoExposeReferenceFrame=on  EllipsoidRadii=[prop_CG_L, prop_CG_L, prop_CG_L/10]  EllipsoidRadiiUnits=m  GraphicEmissiveColor=[0.0 0.0 0.0 1.0]  ExportEntireGeometry=off  SerializedFrames=<Frames/>  MarkerShape=Sphere  MarkerSize=10  GraphicType=FromGeometry  InertiaType=Custom  Mass=air_mass_0  MassUnits=kg  MomentsOfInertia=Iair_xx_yy_zz  MomentsOfInertiaUnits=kg*m^2  GraphicOpacity=1.0  ProductsOfInertia=Iair_yz_zx_xy  ProductsOfInertiaUnits=kg*m^2  GraphicShininess=75  GraphicSpecularColor=[0.5 0.5 0.5 1.0]  GraphicVisPropType=SimpleVisualProperties
      settings: SourceProductBaseCode=MS
      settings: AttributesFormatString=|
      | %<Mass>
      | %<MomentsOfInertia>
      | %<ProductsOfInertia>
  Ground : Ground
  Ground1 : Ground
  Mechanism Configuration : sm_lib/Utilities/Mechanism Configuration  UniformGravity=Constant  GravityVector=[0, 0, -g_const]  GravityUnits=m/s^2  LinearizationDelta=0.001  JointModeTransitionNonlinearIterations=2
  Mux : Mux  Inputs=3
  Mux1 : Mux  Inputs=3
  Product : Product  Multiplication=Matrix(*)
  Propellers : Subsystem
  Reshape2 : Reshape  OutputDimensionality=Column vector (2-D)
  Reshape3 : Reshape  OutputDimensionality=Column vector (2-D)
  Reshape5 : Reshape  OutputDimensionality=Column vector (2-D)
  Signal Specification2 : SignalSpecification  Dimensions=[4,1]
  Solver Configuration : nesl_utility/Solver Configuration  PhysicalDomain=network_engine_domain  SubClassName=solver  LeftPortType=input  RightPortType=generic  Tones=[]  Harmonics=[]  SimulateNoise=off  Profile=off  UseLocalSampling=off  EnableSwitchedLinearOptims=on  FrequencyDomain=off  UseCCode=off  RelTol=0.001  AbsTol=1e-06  MinStep=1e-09  ToWorkspace=off  RevertToSquareIcSolve=off  NumHomotopyIterations=100  PhasorMode=off  PhasorModeNumHarmonics=1  DoDC=off  ResidualTolerance=1e-09  UseLocalSolver=off  LocalSolverChoice=NE_BACKWARD_EULER_ADVANCER  LocalSolverSampleTime=0.001  DoFixedCost=off  MaxNonlinIter=3  MaxModeIter=2  ComputeImpulses=off  ImpulseIterations=2  LinearAlgebra=Sparse  EquationFormulation=NE_TIME_EF  DelaysMemoryBudget=1024  AutomaticFiltering=on  FilteringTimeConstant=0.001  PartitionStorageMethod=AS_NEEDED  PartitionMemoryBudget=1024  PartitionMethod=FAST
      settings: SourceProductBaseCode=PW,SS
  World Frame : sm_lib/Frames and Transforms/World Frame
  echo_MASK_params : Subsystem
  WORLD : PMIOPort  Side=Left
  Ve : Outport  VectorParamsAs1DForOutWhenUnconnected=off
  Xe : Outport  Port=2  VectorParamsAs1DForOutWhenUnconnected=off
  Euler : Outport  Port=3  VectorParamsAs1DForOutWhenUnconnected=off
  bRg (DCM) : Outport  Port=4  VectorParamsAs1DForOutWhenUnconnected=off
  Vb : Outport  Port=5  VectorParamsAs1DForOutWhenUnconnected=off
  p,q,r : Outport  Port=6  VectorParamsAs1DForOutWhenUnconnected=off
  pdot,qdot,rdot : Outport  Port=7  VectorParamsAs1DForOutWhenUnconnected=off
  Ab : Outport  Port=8  VectorParamsAs1DForOutWhenUnconnected=off
  Euler_rates : Outport  Port=9  VectorParamsAs1DForOutWhenUnconnected=off
  Prop_Bus : Outport  Port=10  VectorParamsAs1DForOutWhenUnconnected=off
  wires:
  Propellers/1(Prop_BUS) -> [prop_bus]
  wMOT/1 -> Reshape5/1
  6DOF_JOINT_SYS/6(Ve) -> [Ve]
  6DOF_JOINT_SYS/4(eul_rates) -> [eul_dot]
  Product/1 -> Vb/1
  [wMOT] -> Propellers/1(mot_speed_vec)
  6DOF_JOINT_SYS/1(wb) -> [wb]
  [eul_dot] -> Euler_rates/1
  Reshape2/1 -> Ab/1
  Ground/1 -> Mux/2, Mux/3, Mux/1
  Reshape5/1 -> Signal Specification2/1
  [eul] -> Euler/1
  [Xe] -> Xe/1
  Mux1/1 -> Reshape3/1
  6DOF_JOINT_SYS/3(eul) -> [eul]
  Mux/1 -> Reshape2/1
  [wb] -> p,q,r/1
  Reshape3/1 -> pdot,qdot,rdot/1
  [prop_bus] -> Prop_Bus/1
  [bRg] -> bRg (DCM)/1
  Signal Specification2/1 -> [wMOT]
  [bRg] -> Product/1
  Ground1/1 -> Mux1/2, Mux1/3, Mux1/1
  [Ve] -> Product/2
  6DOF_JOINT_SYS/2(bRg) -> [bRg]
  6DOF_JOINT_SYS/5(Xe) -> [Xe]
  [Ve] -> Ve/1
  connections:
  Solver Configuration/RConn1 -- WORLD/RConn1 -- Mechanism Configuration/RConn1 -- World Frame/RConn1 -- 6DOF_JOINT_SYS/LConn1
  Airframe/RConn1 -- Propellers/LConn1 -- 6DOF_JOINT_SYS/RConn1

== system bh_compare_SM_vs_HAND_quad_and_spin_props/SAR/XYZ_CMDS ==
  Demux : Demux  Tag=STV Demux  Outputs=3
      settings: DisplayOption=none
  FromWs : FromWorkspace  Tag=STV FromWs  VariableName=tuvar
      SigBuilderData=|
      | common.afterFinalStr = 'Extrapolate'
      | common.sampleTime = 0
      | dataSet(1).timeRange = [0 200]
      | dataSet(1).name = 'small_steps'
      | dataSet(2).timeRange = [0 200]
      | dataSet(2).name = 'zStairs_xyConstVEL'
      | dataSet(3).timeRange = [0 500]
      | dataSet(3).name = 'sineWaves'
      | dataSet(4).timeRange = [0 200]
      | dataSet(4).name = 'ZERO'
      | dataSet(5).timeRange = [0 200]
      | dataSet(5).name = 'SEARCH_P1'
      | sbobj.Name = 'Signal Builder'
      | sbobj.Groups(1).Name = 'small_steps'
      | sbobj.Groups(1).Signals(1).Name = 'Z'
      | sbobj.Groups(1).Signals(1).XData = [0 10 10.000001 20 20.000001 30 30.000001 55 200]
      | sbobj.Groups(1).Signals(1).YData = [0 0 2 2 2 2 2 2 2]
      | sbobj.Groups(1).Signals(2).Name = 'X'
      | sbobj.Groups(1).Signals(2).XData = [0 10 10.000001 20 20.000001 30 30.000001 55 200]
      | sbobj.Groups(1).Signals(2).YData = [0 0 0 0 3 3 3 3 3]
      | sbobj.Groups(1).Signals(3).Name = 'Y'
      | sbobj.Groups(1).Signals(3).XData = [0 10 10.000001 20 20.000001 30 30.000001 55 200]
      | sbobj.Groups(1).Signals(3).YData = [0 0 0 0 0 0 1 1 1]
      | sbobj.Groups(1).TimeRange = [0 200]
      | sbobj.Groups(2).Name = 'zStairs_xyConstVEL'
      | sbobj.Groups(2).Signals(1).Name = 'Z'
      | sbobj.Groups(2).Signals(1).XData = [0 10 10.000001 20 20.000001 30 30.000001 40 40.000001 55 200]
      | sbobj.Groups(2).Signals(1).YData = [0 0 1 1 2 2 1 1 0 0 0]
      | sbobj.Groups(2).Signals(2).Name = 'X'
      | sbobj.Groups(2).Signals(2).XData = [0 10 10.000001 20 20.000001 30 30.000001 40 40.000001 55 200]
      | sbobj.Groups(2).Signals(2).YData = [0 1 1.0000001 2 2.0000001 3 3.0000001 4 4.0000001 5.5 20]
      | sbobj.Groups(2).Signals(3).Name = 'Y'
      | sbobj.Groups(2).Signals(3).XData = [0 10 10.000001 20 20.000001 30 30.000001 40 40.000001 55 200]
      | sbobj.Groups(2).Signals(3).YData = [0 0.5 0.50000005 1 1.00000005 1.5 1.50000005 2 2.00000005 2.75 10]
      | sbobj.Groups(2).TimeRange = [0 200]
      | sbobj.Groups(3).Name = 'sineWaves'
      | sbobj.Groups(3).Signals(1).Name = 'Z'
      | sbobj.Groups(3).Signals(1).XData = [0 0.1 0.2 0.3 0.4 0.5 0.6 0.7 0.8 0.9 1 1.1 ... (5001 elements, 1x5001)]
      | sbobj.Groups(3).Signals(1).YData = [0 0.0314107325553 0.0627904665622 0.0941082340641 0.125333128258 0.156434333994 0.18738115819 0.218143060119 0.248689681547 0.278990876699 0.309016742004 0.338737645607 ... (5001 elements, 1x5001)]
      | sbobj.Groups(3).Signals(2).Name = 'X'
      | sbobj.Groups(3).Signals(2).XData = [0 0.1 0.2 0.3 0.4 0.5 0.6 0.7 0.8 0.9 1 1.1 ... (5001 elements, 1x5001)]
      | sbobj.Groups(3).Signals(2).YData = [0 0.01 0.02 0.03 0.04 0.05 0.06 0.07 0.08 0.09 0.1 0.11 ... (5001 elements, 1x5001)]
      | sbobj.Groups(3).Signals(3).Name = 'Y'
      | sbobj.Groups(3).Signals(3).XData = [0 0.1 0.2 0.3 0.4 0.5 0.6 0.7 0.8 0.9 1 1.1 ... (5001 elements, 1x5001)]
      | sbobj.Groups(3).Signals(3).YData = [0 0.0157073040455 0.0314107325553 0.04710641095 0.0627904665622 0.0784590295926 0.0941082340641 0.109734218776 0.125333128258 0.140901113717 0.156434333994 0.171928956505 ... (5001 elements, 1x5001)]
      | sbobj.Groups(3).TimeRange = [0 500]
      | sbobj.Groups(4).Name = 'ZERO'
      | sbobj.Groups(4).Signals(1).Name = 'Z'
      | sbobj.Groups(4).Signals(1).XData = [0 200]
      | sbobj.Groups(4).Signals(1).YData = [0 0]
      | sbobj.Groups(4).Signals(2).Name = 'X'
      | sbobj.Groups(4).Signals(2).XData = [0 200]
      | sbobj.Groups(4).Signals(2).YData = [0 0]
      | sbobj.Groups(4).Signals(3).Name = 'Y'
      | sbobj.Groups(4).Signals(3).XData = [0 200]
      | sbobj.Groups(4).Signals(3).YData = [0 0]
      | sbobj.Groups(4).TimeRange = [0 200]
      | sbobj.Groups(5).Name = 'SEARCH_P1'
      | sbobj.Groups(5).Signals(1).Name = 'Z'
      | sbobj.Groups(5).Signals(1).XData = [0 7 27 32 52 57 77 82 102 107 127 132 157 187 200]
      | sbobj.Groups(5).Signals(1).YData = [0 5 5 5 5 5 5 5 5 5 5 5 5 0 0]
      | sbobj.Groups(5).Signals(2).Name = 'X'
      | sbobj.Groups(5).Signals(2).XData = [0 7 27 32 52 57 77 82 102 107 127 132 157 187 200]
      | sbobj.Groups(5).Signals(2).YData = [0 5 25 25 5 5 25 25 5 5 25 25 0 0 0]
      | sbobj.Groups(5).Signals(3).Name = 'Y'
      | sbobj.Groups(5).Signals(3).XData = [0 7 27 32 52 57 77 82 102 107 127 132 157 187 200]
      | sbobj.Groups(5).Signals(3).YData = [0 5 5 10 10 15 15 20 20 25 25 30 30 0 0]
      | sbobj.Groups(5).TimeRange = [0 200]
  Z : Outport  VectorParamsAs1DForOutWhenUnconnected=off
  X : Outport  Tag=STV Outport  Port=2  VectorParamsAs1DForOutWhenUnconnected=off
  Y : Outport  Tag=STV Outport  Port=3  VectorParamsAs1DForOutWhenUnconnected=off
  wires:
  Demux/1 -> Z/1
  FromWs/1 -> Demux/1
  Demux/2 -> X/1
  Demux/3 -> Y/1

== system bh_compare_SM_vs_HAND_quad_and_spin_props/XYZ CMD_LIMITS1/prefilter ==
  note: Y = U *     wn^2/( s^2 + 2*p*wn*s + wn^2)
      | Y*( s^2 + 2*p*wn*s + wn^2) = U * wn^2
      |
      | y'' + y'*2*p*wn + y*wn^2 = U*wn^2
  U : Inport
  Gain : Gain  Gain=2*p*wn
  Gain1 : Gain  Gain=wn^2
  Gain2 : Gain  Gain=wn^2
  Integrator : Integrator
  Integrator1 : Integrator
  Sum : Sum  Inputs=|+--
  U_filt : Outport  VectorParamsAs1DForOutWhenUnconnected=off
  U_DOT : Outport  Port=2  VectorParamsAs1DForOutWhenUnconnected=off
  wires:
  Integrator/1 -> Integrator1/1, [Y_DOT], Gain/1  "y_dot"
  Sum/1 -> Integrator/1  "y_dot_dot"
  Integrator1/1 -> Gain1/1, U_filt/1  "y"
  U/1 -> Gain2/1
  Gain2/1 -> Sum/1
  Gain/1 -> Sum/3
  Gain1/1 -> Sum/2
  [Y_DOT] -> U_DOT/1

== system bh_compare_SM_vs_HAND_quad_and_spin_props/a_circle1/Signal Builder ==
  Demux : Demux  Tag=STV Demux  Outputs=2
      settings: DisplayOption=none
  FromWs : FromWorkspace  Tag=STV FromWs  VariableName=tuvar
      SigBuilderData=|
      | common.afterFinalStr = 'Extrapolate'
      | common.sampleTime = 0
      | dataSet.timeRange = [0 22]
      | dataSet.name = 'Group 1'
      | sbobj.Groups.Name = 'Group 1'
      | sbobj.Groups.Signals(1).Name = 'Signal 1'
      | sbobj.Groups.Signals(1).XData = [0 7.95 7.95 22]
      | sbobj.Groups.Signals(1).YData = [0 0 1.99 1.98]
      | sbobj.Groups.Signals(2).Name = 'Signal 2'
      | sbobj.Groups.Signals(2).XData = [0 12 16 22]
      | sbobj.Groups.Signals(2).YData = [0 0 1 1]
      | sbobj.Groups.TimeRange = [0 22]
  Signal 1 : Outport  Tag=STV Outport  VectorParamsAs1DForOutWhenUnconnected=off
  Signal 2 : Outport  Tag=STV Outport  Port=2  VectorParamsAs1DForOutWhenUnconnected=off
  wires:
  Demux/1 -> Signal 1/1
  FromWs/1 -> Demux/1
  Demux/2 -> Signal 2/1

== system bh_compare_SM_vs_HAND_quad_and_spin_props/a_circle1/Subsystem ==
  RPS : Inport
  Constant : Constant  Value=2*pi
  Product : Product  Inputs=**
  w_rad_psec : Outport  VectorParamsAs1DForOutWhenUnconnected=off
  wires:
  Constant/1 -> Product/2
  RPS/1 -> Product/1
  Product/1 -> w_rad_psec/1

== system bh_compare_SM_vs_HAND_quad_and_spin_props/CONT_SYS Force_Moment_CMDS/PITCH_and_ROLL_CONT/Apply Pitch and Roll Saturation Limits ==
  In1 : Inport
  Degrees to Radians : simulink_extras/Transformations/Degrees to Radians
  Radians to Degrees : simulink_extras/Transformations/Radians to Degrees
  Saturation : Saturate  UpperLimit=P_veh.LIMITS_tilt_max_deg  LowerLimit=-1*P_veh.LIMITS_tilt_max_deg
      settings: AttributesFormatString=|
      | MAX =    %<UpperLimit>
      | MIN = %<LowerLimit>
  Out1 : Outport  VectorParamsAs1DForOutWhenUnconnected=off
  wires:
  In1/1 -> Radians to Degrees/1
  Saturation/1 -> Degrees to Radians/1
  Radians to Degrees/1 -> Saturation/1
  Degrees to Radians/1 -> Out1/1

== system bh_compare_SM_vs_HAND_quad_and_spin_props/CONT_SYS Force_Moment_CMDS/PITCH_and_ROLL_CONT/FINAL_DES_PITCH_CONTROL ==
  note: NOTE: 1 radian = 57 degrees
  ANG_CMD : Inport
  ANG_MEAS : Inport  Port=2
  ANG_dot_MEAS : Inport  Port=3
  P_CONT : slpidlib/PID Controller  Controller=P  Form=Parallel  TimeDomain=Continuous-time  UseExternalTs=off  SampleTime=-1  IntegratorMethod=Forward Euler  FilterMethod=Forward Euler  ControllerParametersSource=internal  P=0.0507941015552232  I=7.09690484808648  D=-0.334898279224841  UseFilter=on  N=17.076664592689  TunerSelectOption=Transfer Function Based (PID Tuner App)  InitialConditionSource=internal  InitialConditionForIntegrator=0  InitialConditionForFilter=0  DifferentiatorICPrevScaledInput=0  ExternalReset=none  TrackingMode=off  Kt=1  LimitOutput=off  SatLimitsSource=internal  UpperSaturationLimit=inf  LowerSaturationLimit=-inf  LinearizeAsGain=on  AntiWindupMode=none  Kb=1  POutMin=[]  POutMax=[]  IOutMin=[]  IOutMax=[]  DOutMin=[]  DOutMax=[]  NOutMin=[]  NOutMax=[]  SumOutMin=[]  SumOutMax=[]  SaturationOutMin=[]  SaturationOutMax=[]  PParamMin=[]  PParamMax=[]  IParamMin=[]  IParamMax=[]  DParamMin=[]  DParamMax=[]  NParamMin=[]  NParamMax=[]  KbParamMin=[]  KbParamMax=[]  KtParamMin=[]  KtParamMax=[]  KbOutMin=[]  KbOutMax=[]  KtOutMin=[]  KtOutMax=[]  IntegratorOutMin=[]  IntegratorOutMax=[]  FilterOutMin=[]  FilterOutMax=[]  SumI1OutMin=[]  SumI1OutMax=[]  SumI2OutMin=[]  SumI2OutMax=[]  SumI3OutMin=[]  SumI3OutMax=[]  SumI4OutMin=[]  SumI4OutMax=[]  SumDOutMin=[]  SumDOutMax=[]  DifferentiatorOutMin=[]  DifferentiatorOutMax=[]  FilterDiffOutCoefMin=[]  FilterDiffOutCoefMax=[]  ReciprocalOutMin=[]  ReciprocalOutMax=[]  SumDenOutMin=[]  SumDenOutMax=[]  SumNumOutMin=[]  SumNumOutMax=[]  DivideOutMin=[]  DivideOutMax=[]  UdiffTsProdOutMin=[]  UdiffTsProdOutMax=[]  NTsProdOutMin=[]  NTsProdOutMax=[]  UintegralTsProdOutMin=[]  UintegralTsProdOutMax=[]  UngainTsProdOutMin=[]  UngainTsProdOutMax=[]  IntegratorContinuousStateAttributes=''  IntegratorStateMustResolveToSignalObject=off  IntegratorRTWStateStorageClass=Auto  FilterContinuousStateAttributes=''  FilterStateMustResolveToSignalObject=off  FilterRTWStateStorageClass=Auto  ParallelPVariant=InternalParameters  IdealPVariant=Disabled  IVariant=Disabled  DVariant=Disabled  IntegratorVariant=Disabled  SatVariant=Disabled  AWVariant=Disabled  PCopyVariant=Disabled  TRVariant=Disabled  FdbkBlocksVariant=Forward  IdealPFdbkVariant=Disabled  SatFdbkVariant=Disabled  DerivativeFilterVariant=Disabled  NVariant=Disabled  NCopyVariant=Disabled_SignalSpec  FilterICVariant=Disabled  IntegratorICVariant=Disabled  ExternalResetVariant=Disabled  TRSumVariant=Passthrough  SumFdbkVariant=Disabled  SumVariant=Passthrough_P  TsampFilterVariant=InternalTs  TsampNgainVariant=Passthrough  TsampIntegralVariant=Disabled_SignalSpec  ExternalSaturationOutDataTypeStr=Inherit: Same as second input
  P_CONT_too : slpidlib/PID Controller  Controller=P  Form=Parallel  TimeDomain=Continuous-time  UseExternalTs=off  SampleTime=-1  IntegratorMethod=Forward Euler  FilterMethod=Forward Euler  ControllerParametersSource=internal  P=3.111442907298  I=0.151389824684851  D=0  UseFilter=on  N=100  TunerSelectOption=Transfer Function Based (PID Tuner App)  InitialConditionSource=internal  InitialConditionForIntegrator=0  InitialConditionForFilter=0  DifferentiatorICPrevScaledInput=0  ExternalReset=none  TrackingMode=off  Kt=1  LimitOutput=off  SatLimitsSource=internal  UpperSaturationLimit=inf  LowerSaturationLimit=-inf  LinearizeAsGain=on  AntiWindupMode=none  Kb=1  POutMin=[]  POutMax=[]  IOutMin=[]  IOutMax=[]  DOutMin=[]  DOutMax=[]  NOutMin=[]  NOutMax=[]  SumOutMin=[]  SumOutMax=[]  SaturationOutMin=[]  SaturationOutMax=[]  PParamMin=[]  PParamMax=[]  IParamMin=[]  IParamMax=[]  DParamMin=[]  DParamMax=[]  NParamMin=[]  NParamMax=[]  KbParamMin=[]  KbParamMax=[]  KtParamMin=[]  KtParamMax=[]  KbOutMin=[]  KbOutMax=[]  KtOutMin=[]  KtOutMax=[]  IntegratorOutMin=[]  IntegratorOutMax=[]  FilterOutMin=[]  FilterOutMax=[]  SumI1OutMin=[]  SumI1OutMax=[]  SumI2OutMin=[]  SumI2OutMax=[]  SumI3OutMin=[]  SumI3OutMax=[]  SumI4OutMin=[]  SumI4OutMax=[]  SumDOutMin=[]  SumDOutMax=[]  DifferentiatorOutMin=[]  DifferentiatorOutMax=[]  FilterDiffOutCoefMin=[]  FilterDiffOutCoefMax=[]  ReciprocalOutMin=[]  ReciprocalOutMax=[]  SumDenOutMin=[]  SumDenOutMax=[]  SumNumOutMin=[]  SumNumOutMax=[]  DivideOutMin=[]  DivideOutMax=[]  UdiffTsProdOutMin=[]  UdiffTsProdOutMax=[]  NTsProdOutMin=[]  NTsProdOutMax=[]  UintegralTsProdOutMin=[]  UintegralTsProdOutMax=[]  UngainTsProdOutMin=[]  UngainTsProdOutMax=[]  IntegratorContinuousStateAttributes=''  IntegratorStateMustResolveToSignalObject=off  IntegratorRTWStateStorageClass=Auto  FilterContinuousStateAttributes=''  FilterStateMustResolveToSignalObject=off  FilterRTWStateStorageClass=Auto  ParallelPVariant=InternalParameters  IdealPVariant=Disabled  IVariant=Disabled  DVariant=Disabled  IntegratorVariant=Disabled  SatVariant=Disabled  AWVariant=Disabled  PCopyVariant=Disabled  TRVariant=Disabled  FdbkBlocksVariant=Forward  IdealPFdbkVariant=Disabled  SatFdbkVariant=Disabled  DerivativeFilterVariant=Disabled  NVariant=Disabled  NCopyVariant=Disabled_SignalSpec  FilterICVariant=Disabled  IntegratorICVariant=Disabled  ExternalResetVariant=Disabled  TRSumVariant=Passthrough  SumFdbkVariant=Disabled  SumVariant=Passthrough_P  TsampFilterVariant=InternalTs  TsampNgainVariant=Passthrough  TsampIntegralVariant=Disabled_SignalSpec  ExternalSaturationOutDataTypeStr=Inherit: Same as second input
  Sum1 : Sum  Inputs=|+-
  Sum3 : Sum  Inputs=|+-
  TQ : Outport  VectorParamsAs1DForOutWhenUnconnected=off
  wires:
  Sum3/1 -> P_CONT/1
  P_CONT/1 -> TQ/1  "TQ"
  ANG_MEAS/1 -> Sum1/2
  ANG_dot_MEAS/1 -> Sum3/2
  Sum1/1 -> P_CONT_too/1
  ANG_CMD/1 -> Sum1/1
  P_CONT_too/1 -> Sum3/1
